simulink model "untitled"  (R2025a)
settings: Solver=VariableStepAuto  StartTime=0.0  StopTime=1  RelTol=1e-3
settings Model: Creator=HyperBook  LastModifiedBy=HyperBook

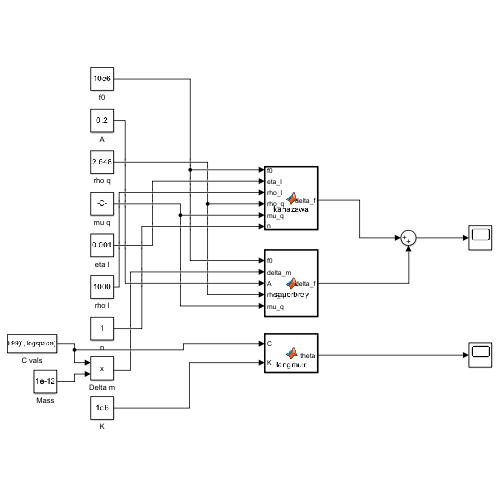
[thumbnail: Simulink's stored preview of the top-level diagram]
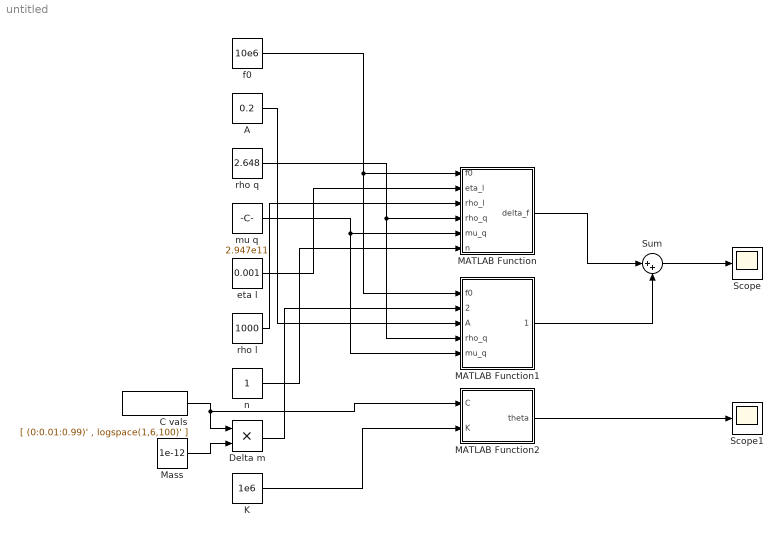
== system untitled ==
  A : Constant  Value=0.2
  C vals : FromWorkspace  VariableName=[ (0:0.01:0.99)' , logspace(1,6,100)' ]
  Delta m : Product
  K : Constant  Value=1e6
  MATLAB Function : MATLAB Function  TreatAsAtomicUnit=on
  MATLAB Function1 : MATLAB Function  TreatAsAtomicUnit=on
  MATLAB Function2 : MATLAB Function  TreatAsAtomicUnit=on
  Mass : Constant  Value=1e-12
  Scope : Scope
      settings: ActiveDisplayYMinimum=-21609.819318745813  ActiveDisplayYMaximum=-20039.471489712181
  Scope1 : Scope
      settings: ActiveDisplayYMinimum=0.999999887500124  ActiveDisplayYMaximum=1.0000000124989852
  Sum : Sum  Inputs=|++
  eta l : Constant  Value=0.001
  f0 : Constant  Value=10e6
  mu q : Constant  Value=2.947e11
  n : Constant
  rho l : Constant  Value=1000
  rho q : Constant  Value=2.648
  wires:
  Mass/1 -> Delta m/2
  f0/1 -> MATLAB Function1/1(f0), MATLAB Function/1(f0)
  eta l/1 -> MATLAB Function/2(eta_l)
  rho l/1 -> MATLAB Function/3(rho_l)
  rho q/1 -> MATLAB Function1/4(rho_q), MATLAB Function/4(rho_q)
  mu q/1 -> MATLAB Function1/5(mu_q), MATLAB Function/5(mu_q)
  n/1 -> MATLAB Function/6(n)
  Delta m/1 -> MATLAB Function1/2(delta_m)
  A/1 -> MATLAB Function1/3(A)
  C vals/1 -> MATLAB Function2/1(C), Delta m/1
  K/1 -> MATLAB Function2/2(K)
  MATLAB Function2/1(theta) -> Scope1/1
  MATLAB Function/1(delta_f) -> Sum/1
  MATLAB Function1/1(delta_f) -> Sum/2
  Sum/1 -> Scope/1

== matlab function untitled/MATLAB Function1 ==
  data: f0 input; delta_f output; delta_m input; A input; rho_q input; mu_q input
function delta_f = sauerbrey(f0, delta_m, A, rho_q, mu_q)
% Równanie Sauerbreya – zmiana częstotliwości w funkcji przyrostu masy
    delta_f = -2 * f0^2 * delta_m / (A * sqrt(rho_q * mu_q));
end

== matlab function untitled/MATLAB Function ==
  data: f0 input; delta_f output; eta_l input; rho_l input; rho_q input; mu_q input; n input
function delta_f = kanazawa(f0, eta_l, rho_l, rho_q, mu_q, n)
% Równanie Kanazawy-Gordona – zmiana częstotliwości w cieczy
    delta_f = -sqrt(n) * f0^(3/2) * sqrt(eta_l * rho_l) / sqrt(pi * rho_q * mu_q);
end

== matlab function untitled/MATLAB Function2 ==
  data: C input; theta output; K input
function theta = langmuir(C, K)
% Model Langmuira – pokrycie powierzchni przez bakterie
    theta = (K * C) / (1 + K * C);
end
